simulink model "problem_41s"  (R2018b)
settings: Solver=FixedStepAuto  StartTime=0.0  StopTime=6  FixedStep=0.001  RelTol=1e-3
settings Model: Creator=HyperDrive  LastModifiedBy=HyperDrive

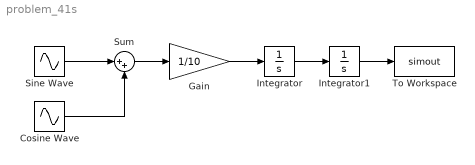
== system problem_41s ==
  Cosine Wave : Sin  Amplitude=5  Frequency=3  Phase=pi/2  SampleTime=0
  Gain : Gain  Gain=1/10
  Integrator : Integrator  InitialCondition=1
  Integrator1 : Integrator  InitialCondition=4
  Sine Wave : Sin  Amplitude=7  Frequency=4  SampleTime=0
  Sum : Sum  Inputs=|++
  To Workspace : ToWorkspace  VariableName=simout  SaveFormat=Timeseries  SampleTime=-1
  wires:
  Cosine Wave/1 -> Sum/2
  Sine Wave/1 -> Sum/1
  Sum/1 -> Gain/1
  Gain/1 -> Integrator/1
  Integrator/1 -> Integrator1/1
  Integrator1/1 -> To Workspace/1
